simulink model "sampleModel1559"  (R2023a)
settings: Solver=VariableStepAuto  StartTime=0.0  StopTime=10.0  RelTol=1e-3
libraries: hdlsllib x7, simulink x4
settings Model: Creator=user1  LastModifiedBy=user1

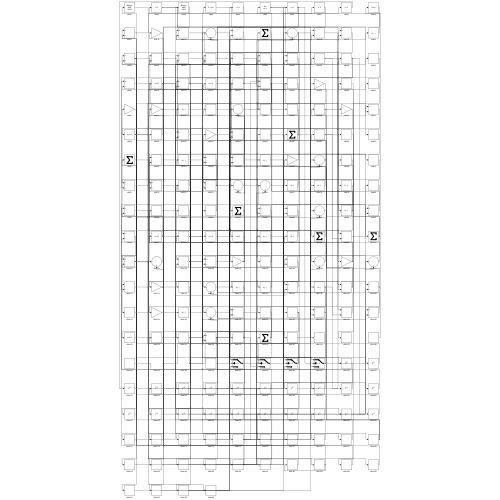
[thumbnail: Simulink's stored preview of the top-level diagram]
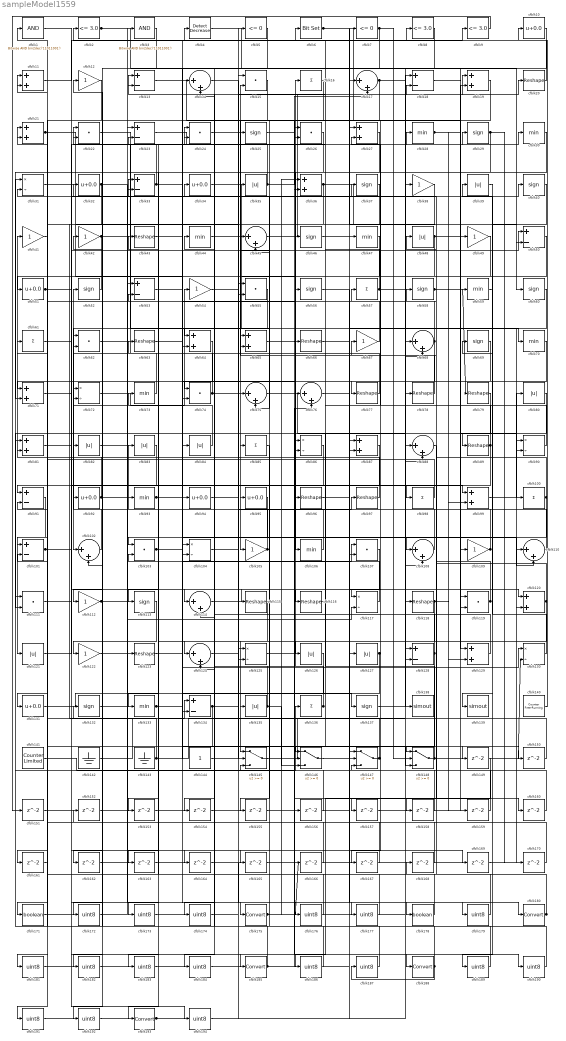
== system sampleModel1559 ==
  cfblk1 : simulink/Logic and Bit Operations/Bitwise Operator  logicop=AND  UseBitMask=on  BitMask=bin2dec('11011001')  BitMaskRealWorld=Stored Integer
      settings: LibrarySourceBlock=|
      | hdlsllib/Logic and Bit
      | Operations/Bitwise
      | Operator
  cfblk{10,32,34,51,92,94..95,131} (8 alike) : Bias  Bias=0.0  SaturateOnIntegerOverflow=off
  cfblk{16,57,61,85,98,100,136} (7 alike) : Sum  Inputs=+
  cfblk{13,18,23,33,50,53,91,101,128,134} (10 alike) : Sum  Inputs=+-
  cfblk{14,17,45,68,75..76,88,102,108,110,114,124} (12 alike) : Sum  Inputs=|++
  cfblk{15,22,24,26,55,62,74,103,107,111,119} (11 alike) : DotProduct  OutDataTypeStr=Inherit: Inherit via internal rule
  cfblk{31,72,86,90,104,117,125,130} (8 alike) : Product  Inputs=*/  RndMeth=Zero  SaturateOnIntegerOverflow=on
  cfblk{12,38,41..42,49,54,67,105,109,112,122} (11 alike) : Gain
  cfblk{28,30,44,47,59,70,73,93,106,133} (10 alike) : MinMax
  cfblk{11,19,21,27,36,64..65,71,81,87,99,120,129} (13 alike) : Sum
  cfblk{25,29,37,40,46,52,56,58,60,69,113,132,137} (13 alike) : Signum
  cfblk{20,43,63,66,77..79,89,96..97,115..116,118,123} (14 alike) : Reshape
  cfblk{35,39,48,80,82..84,121,126..127,135} (11 alike) : Abs  SaturateOnIntegerOverflow=off
  cfblk138 : ToWorkspace  VariableName=simout  SaveFormat=Timeseries  SampleTime=-1
  cfblk139 : ToWorkspace  VariableName=simout  SaveFormat=Timeseries  SampleTime=-1
  cfblk140 : hdlsllib/Sources/Counter Free-Running  NumBits=16  tsamp=-1
  cfblk141 : hdlsllib/Sources/Counter Limited  uplimit=7  tsamp=-1
  cfblk142 : Ground
  cfblk143 : Ground
  cfblk144 : Constant  SampleTime=-1
  cfblk{145..148} (4 alike) : Switch  SaturateOnIntegerOverflow=off  InputSameDT=off
  cfblk{149..170} (22 alike) : Delay  SampleTime=1
  cfblk171 : DataTypeConversion  OutDataTypeStr=boolean  SaturateOnIntegerOverflow=off  RndMeth=Floor
  cfblk{172..174,176..177,179,181..184,186..187,189..192,194} (17 alike) : DataTypeConversion  OutDataTypeStr=uint8  SaturateOnIntegerOverflow=off  RndMeth=Floor
  cfblk{175,180,185,188,193} (5 alike) : DataTypeConversion  SaturateOnIntegerOverflow=off  RndMeth=Floor
  cfblk178 : DataTypeConversion  OutDataTypeStr=boolean  SaturateOnIntegerOverflow=off  RndMeth=Floor
  cfblk2 : hdlsllib/Logic and Bit Operations/Compare To Constant  relop=<=  const=3.0  OutDataTypeStr=boolean
  cfblk3 : simulink/Logic and Bit Operations/Bitwise Operator  logicop=AND  UseBitMask=on  BitMask=bin2dec('11011001')  BitMaskRealWorld=Stored Integer
      settings: LibrarySourceBlock=|
      | hdlsllib/Logic and Bit
      | Operations/Bitwise
      | Operator
  cfblk4 : simulink/Logic and Bit Operations/Detect Decrease  vinit=0.0  OutDataTypeStr=boolean
      settings: LibrarySourceBlock=|
      | hdlsllib/Logic and Bit
      | Operations/Detect
      | Decrease
  cfblk5 : hdlsllib/Logic and Bit Operations/Compare To Zero  relop=<=  OutDataTypeStr=boolean
  cfblk6 : simulink/Logic and Bit Operations/Bit Set  iBit=0
      settings: LibrarySourceBlock=|
      | hdlsllib/Logic and Bit
      | Operations/Bit Set
  cfblk7 : hdlsllib/Logic and Bit Operations/Compare To Zero  relop=<=  OutDataTypeStr=boolean
  cfblk8 : hdlsllib/Logic and Bit Operations/Compare To Constant  relop=<=  const=3.0  OutDataTypeStr=boolean
  cfblk9 : hdlsllib/Logic and Bit Operations/Compare To Constant  relop=<=  const=3.0  OutDataTypeStr=boolean
  wires:
  cfblk105/1 -> cfblk52/1, cfblk45/1
  cfblk53/1 -> cfblk175/1
  cfblk45/1 -> cfblk20/1
  cfblk73/1 -> cfblk24/1
  cfblk120/1 -> cfblk67/1, cfblk146/1
  cfblk91/1 -> cfblk121/1
  cfblk72/1 -> cfblk54/1
  cfblk17/1 -> cfblk105/1, cfblk65/1, cfblk36/2, cfblk68/2
  cfblk108/1 -> cfblk83/1
  cfblk118/1 -> cfblk145/1, cfblk159/1
  cfblk146/1 -> cfblk47/1
  cfblk34/1 -> cfblk70/1
  cfblk27/1 -> cfblk133/1
  cfblk58/1 -> cfblk79/1, cfblk129/2
  cfblk106/1 -> cfblk73/1
  cfblk129/1 -> cfblk63/1
  cfblk32/1 -> cfblk134/1, cfblk119/2, cfblk164/1
  cfblk140/1 -> cfblk2/1
  cfblk136/1 -> cfblk16/1, cfblk103/2
  cfblk130/1 -> cfblk39/1
  cfblk8/1 -> cfblk64/1
  cfblk10/1 -> cfblk112/1
  cfblk133/1 -> cfblk9/1, cfblk130/1
  cfblk55/1 -> cfblk102/1
  cfblk22/1 -> cfblk100/1
  cfblk109/1 -> cfblk93/1, cfblk45/2
  cfblk40/1 -> cfblk89/1
  cfblk39/1 -> cfblk139/1
  cfblk26/1 -> cfblk106/1
  cfblk56/1 -> cfblk127/1
  cfblk97/1 -> cfblk41/1
  cfblk128/1 -> cfblk32/1, cfblk191/1
  cfblk57/1 -> cfblk118/1, cfblk26/2
  cfblk13/1 -> cfblk59/1
  cfblk131/1 -> cfblk137/1
  cfblk132/1 -> cfblk123/1
  cfblk100/1 -> cfblk69/1, cfblk31/2, cfblk153/1
  cfblk101/1 -> cfblk114/1, cfblk169/1
  cfblk114/1 -> cfblk120/1
  cfblk102/1 -> cfblk62/1
  cfblk23/1 -> cfblk29/1
  cfblk16/1 -> cfblk95/1
  cfblk31/1 -> cfblk94/1
  cfblk77/1 -> cfblk12/1
  cfblk52/1 -> cfblk51/1
  cfblk50/1 -> cfblk117/1
  cfblk141/1 -> cfblk136/1
  cfblk90/1 -> cfblk13/1
  cfblk94/1 -> cfblk19/1
  cfblk24/1 -> cfblk85/1
  cfblk104/1 -> cfblk30/1
  cfblk30/1 -> cfblk72/1
  cfblk69/1 -> cfblk113/1
  cfblk67/1 -> cfblk44/1
  cfblk43/1 -> cfblk14/1
  cfblk80/1 -> cfblk126/1
  cfblk35/1 -> cfblk24/2, cfblk17/2
  cfblk126/1 -> cfblk134/2
  cfblk71/1 -> cfblk34/1
  cfblk7/1 -> cfblk64/2, cfblk14/2, cfblk148/2
  cfblk20/1 -> cfblk10/1
  cfblk4/1 -> cfblk88/1
  cfblk36/1 -> cfblk119/1, cfblk75/2, cfblk171/1
  cfblk62/1 -> cfblk28/1
  cfblk107/1 -> cfblk147/2
  cfblk78/1 -> cfblk15/2
  cfblk12/1 -> cfblk101/1
  cfblk112/1 -> cfblk72/2, cfblk176/1
  cfblk98/1 -> cfblk21/1
  cfblk11/1 -> cfblk4/1
  cfblk63/1 -> cfblk135/1
  cfblk18/1 -> cfblk49/1
  cfblk37/1 -> cfblk46/1
  cfblk51/1 -> cfblk25/1, cfblk99/1
  cfblk19/1 -> cfblk77/1
  cfblk103/1 -> cfblk56/1, cfblk37/1
  cfblk84/1 -> cfblk62/2
  cfblk144/1 -> cfblk75/1
  cfblk64/1 -> cfblk131/1
  cfblk66/1 -> cfblk108/1
  cfblk99/1 -> cfblk80/1
  cfblk135/1 -> cfblk13/2, cfblk146/3
  cfblk82/1 -> cfblk40/1
  cfblk122/1 -> cfblk117/2
  cfblk47/1 -> cfblk74/1
  cfblk46/1 -> cfblk8/1
  cfblk38/1 -> cfblk193/1
  cfblk96/1 -> cfblk180/1
  cfblk148/1 -> cfblk86/1, cfblk130/2
  cfblk137/1 -> cfblk108/2
  cfblk15/1 -> cfblk122/1
  cfblk2/1 -> cfblk60/1, cfblk129/1
  cfblk61/1 -> cfblk188/1
  cfblk134/1 -> cfblk5/1, cfblk18/2, cfblk163/1
  cfblk119/1 -> cfblk57/1, cfblk65/2
  cfblk25/1 -> cfblk86/2
  cfblk6/1 -> cfblk138/1, cfblk50/2
  cfblk74/1 -> cfblk42/1, cfblk98/1
  cfblk89/1 -> cfblk104/2, cfblk27/2, cfblk22/1
  cfblk5/1 -> cfblk124/1
  cfblk48/1 -> cfblk109/1, cfblk103/1
  cfblk123/1 -> cfblk107/1
  cfblk68/1 -> cfblk11/2, cfblk157/1
  cfblk83/1 -> cfblk91/1
  cfblk116/1 -> cfblk6/1
  cfblk127/1 -> cfblk167/1, cfblk184/1
  cfblk117/1 -> cfblk43/1
  cfblk143/1 -> cfblk84/1, cfblk88/2, cfblk91/2
  cfblk21/1 -> cfblk145/2, cfblk181/1
  cfblk60/1 -> cfblk107/2
  cfblk145/1 -> cfblk7/1
  cfblk124/1 -> cfblk97/1
  cfblk14/1 -> cfblk148/1
  cfblk92/1 -> cfblk11/1, cfblk165/1
  cfblk75/1 -> cfblk128/1
  cfblk147/1 -> cfblk33/1, cfblk23/2
  cfblk29/1 -> cfblk71/2, cfblk128/2, cfblk170/1
  cfblk42/1 -> cfblk26/1, cfblk71/1
  cfblk142/1 -> cfblk74/2
  cfblk28/1 -> cfblk90/2, cfblk99/2
  cfblk93/1 -> cfblk116/1, cfblk148/3
  cfblk44/1 -> cfblk66/1
  cfblk81/1 -> cfblk185/1
  cfblk79/1 -> cfblk111/2
  cfblk121/1 -> cfblk50/1
  cfblk110/1 -> cfblk82/1
  cfblk33/1 -> cfblk76/1, cfblk110/2, cfblk22/2
  cfblk76/1 -> cfblk149/1
  cfblk54/1 -> cfblk150/1
  cfblk150/1 -> cfblk104/1
  cfblk9/1 -> cfblk151/1
  cfblk151/1 -> cfblk27/1
  cfblk152/1 -> cfblk55/1
  cfblk153/1 -> cfblk33/2
  cfblk86/1 -> cfblk154/1
  cfblk154/1 -> cfblk147/1
  cfblk85/1 -> cfblk155/1
  cfblk156/1 -> cfblk111/1
  cfblk157/1 -> cfblk19/2
  cfblk88/1 -> cfblk158/1
  cfblk158/1 -> cfblk114/2
  cfblk159/1 -> cfblk31/1
  cfblk65/1 -> cfblk160/1
  cfblk160/1 -> cfblk147/3
  cfblk41/1 -> cfblk161/1
  cfblk161/1 -> cfblk21/2
  cfblk49/1 -> cfblk162/1
  cfblk162/1 -> cfblk18/1
  cfblk163/1 -> cfblk120/2
  cfblk165/1 -> cfblk90/1
  cfblk166/1 -> cfblk146/2
  cfblk167/1 -> cfblk102/2
  cfblk168/1 -> cfblk101/2
  cfblk169/1 -> cfblk110/1
  cfblk170/1 -> cfblk23/1
  cfblk171/1 -> cfblk3/1
  cfblk3/1 -> cfblk172/1
  cfblk172/1 -> cfblk92/1
  cfblk115/1 -> cfblk173/1
  cfblk173/1 -> cfblk15/1
  cfblk95/1 -> cfblk174/1
  cfblk174/1 -> cfblk115/1
  cfblk175/1 -> cfblk166/1, cfblk36/1, cfblk68/1, cfblk78/1
  cfblk176/1 -> cfblk53/1
  cfblk164/1 -> cfblk177/1
  cfblk177/1 -> cfblk53/2
  cfblk155/1 -> cfblk178/1
  cfblk178/1 -> cfblk1/1
  cfblk1/1 -> cfblk179/1
  cfblk179/1 -> cfblk58/1
  cfblk180/1 -> cfblk168/1, cfblk145/3, cfblk48/1
  cfblk181/1 -> cfblk96/1
  cfblk87/1 -> cfblk182/1
  cfblk182/1 -> cfblk156/1
  cfblk70/1 -> cfblk183/1
  cfblk183/1 -> cfblk87/1
  cfblk184/1 -> cfblk87/2
  cfblk185/1 -> cfblk124/2, cfblk76/2, cfblk132/1
  cfblk149/1 -> cfblk186/1
  cfblk186/1 -> cfblk81/1
  cfblk187/1 -> cfblk81/2
  cfblk188/1 -> cfblk187/1, cfblk35/1
  cfblk59/1 -> cfblk189/1
  cfblk189/1 -> cfblk61/1
  cfblk125/1 -> cfblk190/1
  cfblk190/1 -> cfblk152/1
  cfblk191/1 -> cfblk125/1
  cfblk113/1 -> cfblk192/1
  cfblk192/1 -> cfblk125/2
  cfblk193/1 -> cfblk17/1, cfblk55/2
  cfblk111/1 -> cfblk194/1
  cfblk194/1 -> cfblk38/1
